simulink model "Function12"  (R2016b)
settings: Solver=VariableStepAuto  StartTime=0.0  StopTime=10.0  RelTol=1e-3
libraries: simulink x2
settings Model: Creator=viett  LastModifiedBy=viett

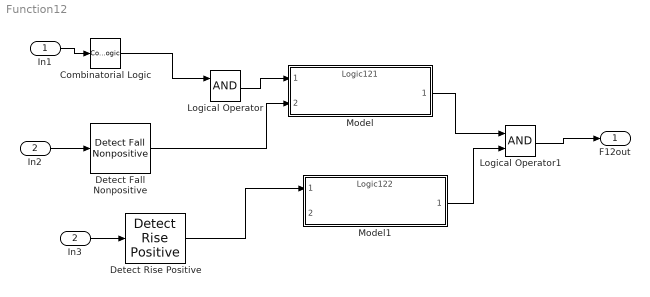
== system Function12 ==
  In1 : Inport
  In2 : Inport  Port=2
  Combinatorial Logic : CombinatorialLogic
  Detect Fall Nonpositive : simulink/Logic and Bit Operations/Detect Fall Nonpositive  vinit=0  OutDataTypeStr=boolean
  Detect Rise Positive : simulink/Logic and Bit Operations/Detect Rise Positive  vinit=0  OutDataTypeStr=boolean
  In3 : InportShadow  Port=2
  Logical Operator : Logic  AllPortsSameDT=off  OutDataTypeStr=boolean
  Logical Operator1 : Logic  AllPortsSameDT=off  OutDataTypeStr=boolean
  Model : ModelReference  ModelNameDialog=Logic121.slx  SimulationMode=Normal  ModelReferenceVersion=1.1
  Model1 : ModelReference  ModelNameDialog=Logic122  SimulationMode=Normal  ModelReferenceVersion=1.1
  F12out : Outport
  wires:
  Logical Operator/1 -> Model/1
  Detect Fall Nonpositive/1 -> Model/2
  Combinatorial Logic/1 -> Logical Operator/1
  Model/1 -> Logical Operator1/1
  Model1/1 -> Logical Operator1/2
  Detect Rise Positive/1 -> Model1/1
  In1/1 -> Combinatorial Logic/1
  In2/1 -> Detect Fall Nonpositive/1
  In3/1 -> Detect Rise Positive/1
  Logical Operator1/1 -> F12out/1
